simulink model "RST_2ordem_prev_vers"  (R2015a)
settings: Solver=ode45  SolverMode=SingleTasking  StartTime=0.0  StopTime=50  RelTol=1e-3
values from neighbouring files (symbols this model uses):
  A = den    [cod_teste_RST_2.m]
  B = num    (= 1)    [cod_teste_RST_2.m]
  ep = 0.6    [cod_teste_RST_2.m]
  R = X(1)    [cod_teste_RST_1.m]    (also in cod_teste_RST_2.m = [1 X(1)])
  S = X(2:end)    [cod_teste_RST_1.m]    (also in cod_teste_RST_2.m = [X(3) X(2)])
  T = sum(PMF)/sum(B)    [cod_teste_RST_1.m]    (also in cod_teste_RST_2.m = sum(Am)/sum(B))
  T_a = 0.1    [cod_teste_RST_2.m]
  Ts = 1    [cod_teste_RST_2.m]
libraries: aerolibutil x1
settings Model: CovMetricSettings=dwe  CovHtmlReporting=off  covSaveCumulativeToWorkspaceVar=off  CovSaveSingleToWorkspaceVar=off  CovExternalEMLEnable=on  Creator=tarci  LastModifiedBy=tarci
settings DataIOCC: LimitDataPoints=off  SaveFormat=Dataset
settings DebuggingCC: SFUnexpectedBacktrackingDiag=error  SFNoUnconditionalDefaultTransitionDiag=error
settings HardwareCC: ProdBitPerPointer=64  ProdLargestAtomicFloat=Float  ProdIntDivRoundTo=Zero  ProdEndianess=LittleEndian  ProdHWDeviceType=Specified
settings ModelReferenceCC: PropagateSignalLabelsOutOfModel=on
settings SFSimCC: SimUseLocalCustomCode=on
settings RTWCC: RTWUseLocalCustomCode=on
settings GRTTargetCC: TargetLangStandard=C99 (ISO)  GeneratePreprocessorConditionals=Use local settings

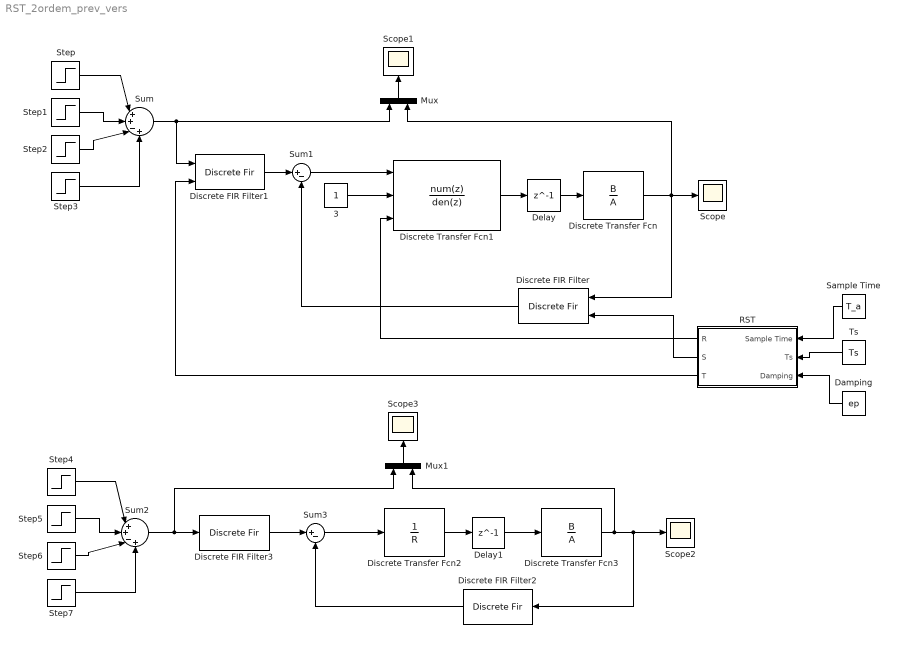
== system RST_2ordem_prev_vers ==
  3 : Constant
  Damping : Constant  Value=ep
  Delay : Delay  DelayLength=1  InitialCondition=0  SampleTime=0.1
  Delay1 : Delay  DelayLength=1  InitialCondition=0  SampleTime=0.1
  Discrete Transfer Fcn : DiscreteTransferFcn  Numerator=B  Denominator=A  SampleTime=0.1
  Discrete Transfer Fcn1 : DiscreteTransferFcn  NumeratorSource=Input port  Numerator=B  DenominatorSource=Input port  Denominator=A  SampleTime=0.1  a0EqualsOne=on
      settings: InputPortMap=u0,p1,p3
  Discrete Transfer Fcn2 : DiscreteTransferFcn  Numerator=1  Denominator=R  SampleTime=0.1
  Discrete Transfer Fcn3 : DiscreteTransferFcn  Numerator=B  Denominator=A  SampleTime=0.1
  Discrete FIR Filter : DiscreteFir  CoefSource=Input port  SampleTime=0.1
  Discrete FIR Filter1 : DiscreteFir  CoefSource=Input port  SampleTime=0.1
  Discrete FIR Filter2 : DiscreteFir  Coefficients=S  SampleTime=0.1
  Discrete FIR Filter3 : DiscreteFir  Coefficients=T  SampleTime=0.1
  Mux : Mux  Inputs=2
  Mux1 : Mux  Inputs=2
  RST : Subsystem
  Sample Time : Constant  Value=T_a
  Scope{,1..3} (4 alike) : Scope
      Scope settings: TimeRange=auto  MaxDataPoints=5000  SaveToWorkspace=off  SaveName=ScopeData  YMin=-0.73435  YMax=6.60919  SampleTime=-1
      Scope1 settings: TimeRange=auto  MaxDataPoints=5000  SaveToWorkspace=off  YMin=-0.73435  YMax=6.60919  SampleTime=-1
      Scope2 settings: TimeRange=auto  MaxDataPoints=5000  SaveToWorkspace=off  SaveName=ScopeData2  YMin=-0.73435  YMax=6.60919  SampleTime=-1
      Scope3 settings: TimeRange=auto  MaxDataPoints=5000  SaveToWorkspace=off  SaveName=ScopeData3  YMin=-0.73435  YMax=6.60919  SampleTime=-1
  Step : Step  SampleTime=0
  Step1 : Step  Time=10  After=3  SampleTime=0
  Step2 : Step  Time=20  After=2  SampleTime=0
  Step3 : Step  Time=30  SampleTime=0
  Step4 : Step  SampleTime=0
  Step5 : Step  Time=10  After=3  SampleTime=0
  Step6 : Step  Time=20  After=2  SampleTime=0
  Step7 : Step  Time=30  SampleTime=0
  Sum : Sum  Inputs=|++-+
  Sum1 : Sum  Inputs=|+-
  Sum2 : Sum  Inputs=|++-+
  Sum3 : Sum  Inputs=|+-
  Ts : Constant  Value=Ts
  wires:
  Step/1 -> Sum/1
  Step1/1 -> Sum/2
  Step2/1 -> Sum/3
  Step3/1 -> Sum/4
  Discrete Transfer Fcn/1 -> Discrete FIR Filter/1, Scope/1, Mux/2
  Delay/1 -> Discrete Transfer Fcn/1
  Sum/1 -> Discrete FIR Filter1/1, Mux/1
  Discrete FIR Filter1/1 -> Sum1/1
  Sum1/1 -> Discrete Transfer Fcn1/1
  Discrete Transfer Fcn1/1 -> Delay/1
  3/1 -> Discrete Transfer Fcn1/2
  Discrete FIR Filter/1 -> Sum1/2
  Mux/1 -> Scope1/1
  RST/1(R) -> Discrete Transfer Fcn1/3
  RST/3(T) -> Discrete FIR Filter1/2
  RST/2(S) -> Discrete FIR Filter/2
  Sample Time/1 -> RST/1(Sample Time)
  Ts/1 -> RST/2(Ts)
  Damping/1 -> RST/3(Damping)
  Step6/1 -> Sum2/3
  Sum3/1 -> Discrete Transfer Fcn2/1
  Delay1/1 -> Discrete Transfer Fcn3/1
  Step7/1 -> Sum2/4
  Discrete Transfer Fcn3/1 -> Scope2/1, Discrete FIR Filter2/1, Mux1/2
  Discrete FIR Filter3/1 -> Sum3/1
  Step4/1 -> Sum2/1
  Step5/1 -> Sum2/2
  Sum2/1 -> Mux1/1, Discrete FIR Filter3/1
  Mux1/1 -> Scope3/1
  Discrete FIR Filter2/1 -> Sum3/2
  Discrete Transfer Fcn2/1 -> Delay1/1

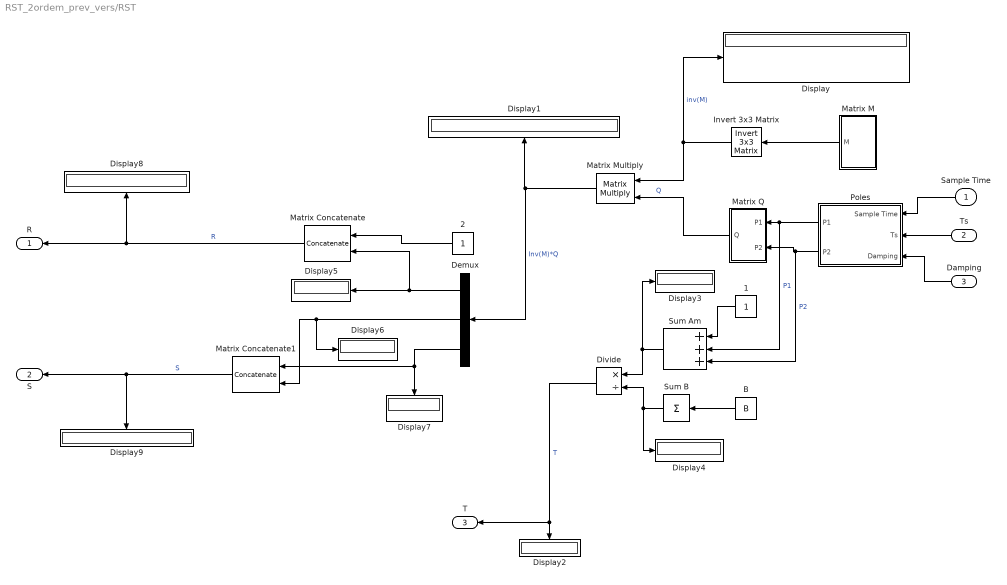
== system RST_2ordem_prev_vers/RST ==
  Sample Time : Inport
  Ts : Inport  Port=2
  Damping : Inport  Port=3
  1 : Constant
  2 : Constant
  B : Constant  Value=B
  Demux : Demux  Outputs=3
  Display{,1..9} (10 alike) : Display
  Divide : Product  Inputs=*/
  Invert 3x3 Matrix : aerolibutil/Invert  3x3 Matrix
  Matrix Concatenate : Concatenate  Mode=Multidimensional array  ConcatenateDimension=2
  Matrix Concatenate1 : Concatenate  Mode=Multidimensional array  ConcatenateDimension=2
  Matrix M : Subsystem
  Matrix Multiply : Product  Multiplication=Matrix(*)
  Matrix Q : Subsystem
  Poles : Subsystem
  Sum Am : Sum  Inputs=+++
  Sum B : Sum  Inputs=+
  R : Outport
  S : Outport  Port=2
  T : Outport  Port=3
  wires:
  Matrix Multiply/1 -> Demux/1, Display1/1  "Inv(M)*Q"
  Demux/1 -> Matrix Concatenate/2, Display5/1
  Sum B/1 -> Divide/2, Display4/1
  Invert 3x3 Matrix/1 -> Matrix Multiply/1, Display/1  "inv(M)"
  Poles/1(P1) -> Sum Am/2, Matrix Q/1(P1)  "P1"
  Matrix Concatenate/1 -> Display8/1, R/1  "R"
  B/1 -> Sum B/1
  Demux/2 -> Display6/1, Matrix Concatenate1/2
  Sum Am/1 -> Divide/1, Display3/1
  Matrix Concatenate1/1 -> S/1, Display9/1  "S"
  Poles/2(P2) -> Sum Am/3, Matrix Q/2(P2)  "P2"
  Divide/1 -> T/1, Display2/1  "T"
  Ts/1 -> Poles/2(Ts)
  Matrix Q/1(Q) -> Matrix Multiply/2  "Q"
  Damping/1 -> Poles/3(Damping)
  Sample Time/1 -> Poles/1(Sample Time)
  1/1 -> Sum Am/1
  Matrix M/1(M) -> Invert 3x3 Matrix/1
  Demux/3 -> Display7/1, Matrix Concatenate1/1
  2/1 -> Matrix Concatenate/1

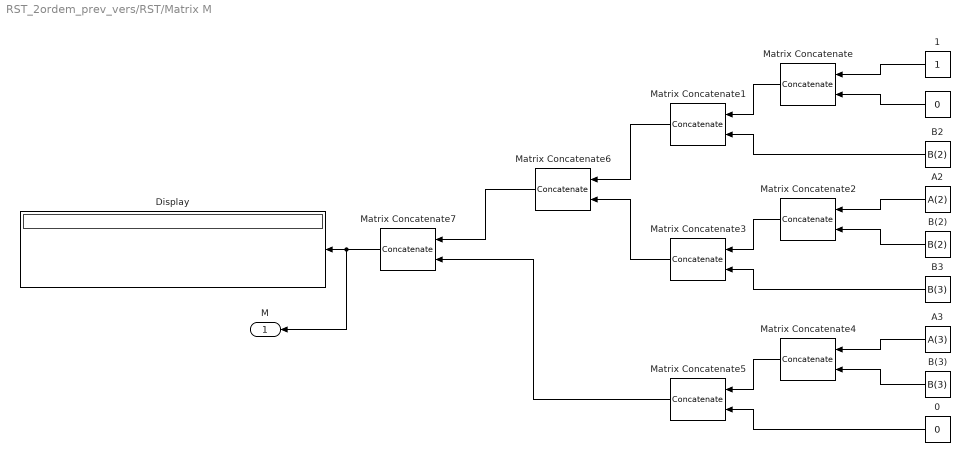
== system RST_2ordem_prev_vers/RST/Matrix M ==
  " " : Constant  Value=0
  " 0" : Constant  Value=0
  " B(2)" : Constant  Value=B(2)
  " B(3)" : Constant  Value=B(3)
  " B2" : Constant  Value=B(2)
  " B3" : Constant  Value=B(3)
  1 : Constant
  A2 : Constant  Value=A(2)
  A3 : Constant  Value=A(3)
  Display : Display
  Matrix Concatenate{,1..5} (6 alike) : Concatenate  Mode=Multidimensional array  ConcatenateDimension=2
  Matrix Concatenate6 : Concatenate  Mode=Multidimensional array
  Matrix Concatenate7 : Concatenate  Mode=Multidimensional array
  M : Outport
  wires:
  " 0"/1 -> Matrix Concatenate5/2
  " "/1 -> Matrix Concatenate/2
  Matrix Concatenate5/1 -> Matrix Concatenate7/2
  1/1 -> Matrix Concatenate/1
  Matrix Concatenate6/1 -> Matrix Concatenate7/1
  Matrix Concatenate7/1 -> M/1, Display/1
  " B(2)"/1 -> Matrix Concatenate2/2
  Matrix Concatenate3/1 -> Matrix Concatenate6/2
  Matrix Concatenate1/1 -> Matrix Concatenate6/1
  Matrix Concatenate/1 -> Matrix Concatenate1/1
  " B2"/1 -> Matrix Concatenate1/2
  " B(3)"/1 -> Matrix Concatenate4/2
  Matrix Concatenate4/1 -> Matrix Concatenate5/1
  A3/1 -> Matrix Concatenate4/1
  Matrix Concatenate2/1 -> Matrix Concatenate3/1
  A2/1 -> Matrix Concatenate2/1
  " B3"/1 -> Matrix Concatenate3/2

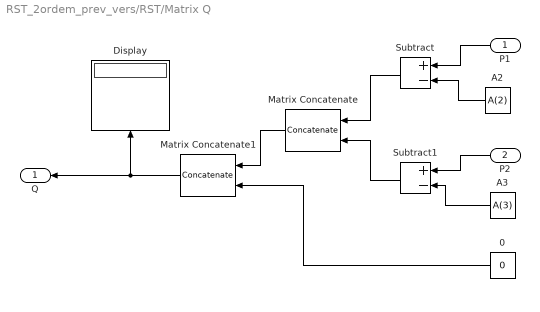
== system RST_2ordem_prev_vers/RST/Matrix Q ==
  P1 : Inport
  P2 : Inport  Port=2
  0 : Constant  Value=0
  A2 : Constant  Value=A(2)
  A3 : Constant  Value=A(3)
  Display : Display
  Matrix Concatenate : Concatenate  Mode=Multidimensional array
  Matrix Concatenate1 : Concatenate  Mode=Multidimensional array
  Subtract : Sum  Inputs=+-
  Subtract1 : Sum  Inputs=+-
  Q : Outport
  wires:
  Subtract1/1 -> Matrix Concatenate/2
  Matrix Concatenate/1 -> Matrix Concatenate1/1
  Subtract/1 -> Matrix Concatenate/1
  A2/1 -> Subtract/2
  Matrix Concatenate1/1 -> Q/1, Display/1
  P1/1 -> Subtract/1
  0/1 -> Matrix Concatenate1/2
  P2/1 -> Subtract1/1
  A3/1 -> Subtract1/2

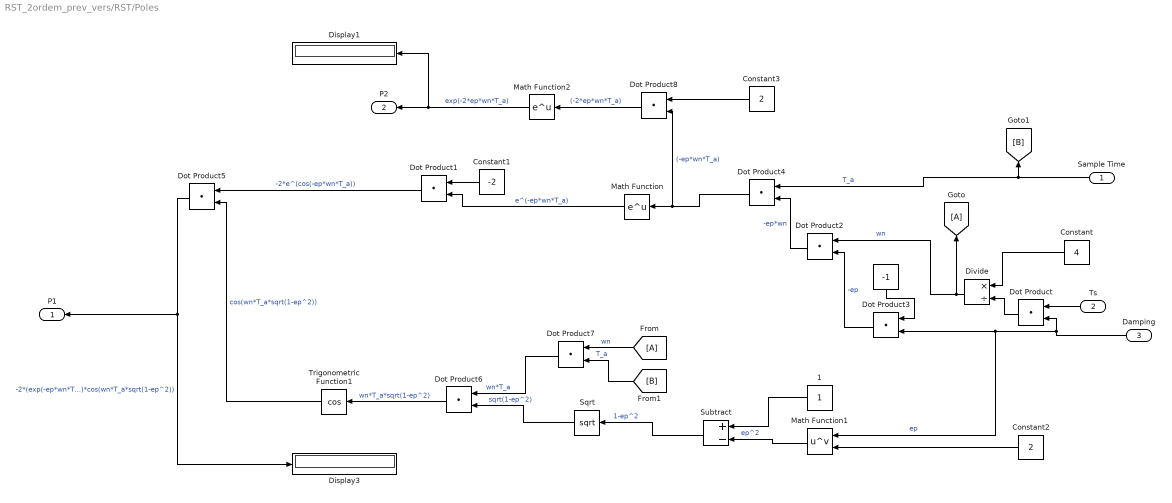
== system RST_2ordem_prev_vers/RST/Poles ==
  Sample Time : Inport
  Ts : Inport  Port=2
  Damping : Inport  Port=3
  " " : Constant  Value=-1
  1 : Constant
  Constant : Constant  Value=4
  Constant1 : Constant  Value=-2
  Constant2 : Constant  Value=2
  Constant3 : Constant  Value=2
  Display1 : Display
  Display3 : Display
  Divide : Product  Inputs=*/
  Dot Product{,1..8} (9 alike) : DotProduct  InputSameDT=on  OutDataTypeStr=Inherit: Inherit via internal rule
  Math Function : Math  SaturateOnIntegerOverflow=on
  Math Function1 : Math  Operator=pow  SaturateOnIntegerOverflow=on
  Math Function2 : Math  SaturateOnIntegerOverflow=on
  Sqrt : Sqrt  SaturateOnIntegerOverflow=on
  Subtract : Sum  Inputs=+-
  Trigonometric Function1 : Trigonometry  Operator=cos
  P1 : Outport
  P2 : Outport  Port=2
  wires:
  Math Function/1 -> Dot Product1/2  "e^(-ep*wn*T_a)"
  Divide/1 -> [A], Dot Product2/1  "wn"
  [A] -> Dot Product7/1  "wn"
  " "/1 -> Dot Product3/1
  Dot Product5/1 -> P1/1, Display3/1  "-2*(exp(-ep*wn*T_a))*cos(wn*T_a*sqrt(1-ep^2))"
  Trigonometric Function1/1 -> Dot Product5/2  "cos(wn*T_a*sqrt(1-ep^2))"
  Ts/1 -> Dot Product/1
  Dot Product/1 -> Divide/2
  Dot Product3/1 -> Dot Product2/2  "-ep"
  Damping/1 -> Math Function1/1, Dot Product3/2, Dot Product/2  "ep"
  Constant/1 -> Divide/1
  Dot Product7/1 -> Dot Product6/1  "wn*T_a"
  Sample Time/1 -> Dot Product4/1, [B]  "T_a"
  Math Function1/1 -> Subtract/2  "ep^2"
  Dot Product1/1 -> Dot Product5/1  "-2*e^(cos(-ep*wn*T_a))"
  Constant2/1 -> Math Function1/2
  1/1 -> Subtract/1
  Constant1/1 -> Dot Product1/1
  Dot Product2/1 -> Dot Product4/2  "-ep*wn"
  [B] -> Dot Product7/2  "T_a"
  Dot Product6/1 -> Trigonometric Function1/1  "wn*T_a*sqrt(1-ep^2)"
  Dot Product4/1 -> Dot Product8/2, Math Function/1  "(-ep*wn*T_a)"
  Sqrt/1 -> Dot Product6/2  "sqrt(1-ep^2)"
  Subtract/1 -> Sqrt/1  "1-ep^2"
  Constant3/1 -> Dot Product8/1
  Dot Product8/1 -> Math Function2/1  "(-2*ep*wn*T_a)"
  Math Function2/1 -> Display1/1, P2/1  "exp(-2*ep*wn*T_a)"
